simulink model "CarModel"  (R2014b)
settings: Solver=ode45  StartTime=0.0  StopTime=10.0  RelTol=1e-3
settings Model: Creator=think  LastModifiedBy=Administrator

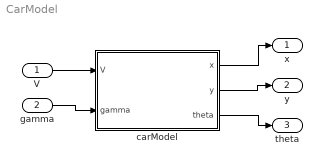
== system CarModel ==
  V : Inport
  gamma : Inport  Port=2
  carModel : Subsystem
  x : Outport
  y : Outport  Port=2
  theta : Outport  Port=3
  wires:
  V/1 -> carModel/1(V)
  gamma/1 -> carModel/2(gamma)
  carModel/1(x) -> x/1
  carModel/2(y) -> y/1
  carModel/3(theta) -> theta/1

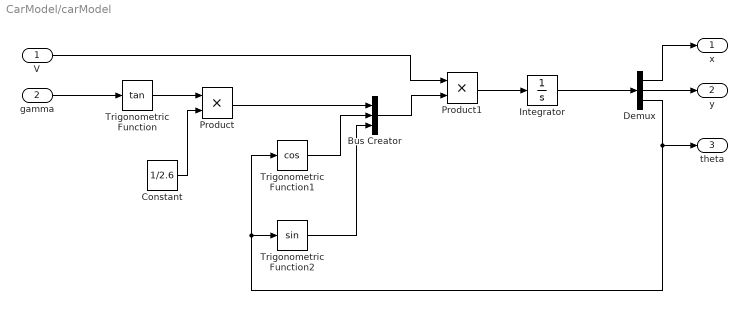
== system CarModel/carModel ==
  V : Inport
  gamma : Inport  Port=2
  Bus Creator : BusCreator  Inputs=3
  Constant : Constant  Value=1/2.6
  Demux : Demux  Outputs=3
  Integrator : Integrator
  Product : Product
  Product1 : Product
  Trigonometric Function : Trigonometry  Operator=tan
  Trigonometric Function1 : Trigonometry  Operator=cos
  Trigonometric Function2 : Trigonometry
  x : Outport
  y : Outport  Port=2
  theta : Outport  Port=3
  wires:
  gamma/1 -> Trigonometric Function/1
  Trigonometric Function1/1 -> Bus Creator/2
  Bus Creator/1 -> Product1/2
  Product1/1 -> Integrator/1
  Demux/2 -> y/1
  Trigonometric Function2/1 -> Bus Creator/3
  Demux/3 -> theta/1, Trigonometric Function1/1, Trigonometric Function2/1
  Product/1 -> Bus Creator/1
  Constant/1 -> Product/2
  Trigonometric Function/1 -> Product/1
  Demux/1 -> x/1
  Integrator/1 -> Demux/1
  V/1 -> Product1/1
